simulink model "Controller"  (R2017b)
settings: Solver=VariableStepAuto  StartTime=0.0  StopTime=200  RelTol=1e-3
settings Model: Creator=Kris  LastModifiedBy=Kris

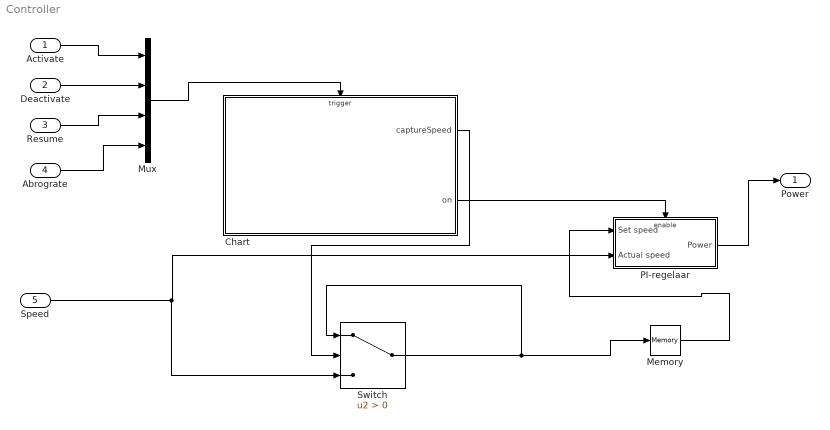
== system Controller ==
  Activate : Inport
  Deactivate : Inport  Port=2
  Resume : Inport  Port=3
  Abrograte : Inport  Port=4
  Speed : Inport  Port=5
  Chart : Stateflow chart  TreatAsAtomicUnit=on
  Memory : Memory
  Mux : Mux
  "PI-regelaar " : Subsystem
  Switch : Switch  Criteria=u2 > Threshold
  Power : Outport
  wires:
  Resume/1 -> Mux/3
  Speed/1 -> Switch/3, "PI-regelaar "/2(Actual speed)
  Chart/2(on) -> "PI-regelaar "/Enable
  Memory/1 -> "PI-regelaar "/1(Set speed)
  Mux/1 -> Chart/Trigger
  Deactivate/1 -> Mux/2
  Chart/1(captureSpeed) -> Switch/2
  "PI-regelaar "/1(Power) -> Power/1
  Abrograte/1 -> Mux/4
  Activate/1 -> Mux/1
  Switch/1 -> Memory/1, Switch/1

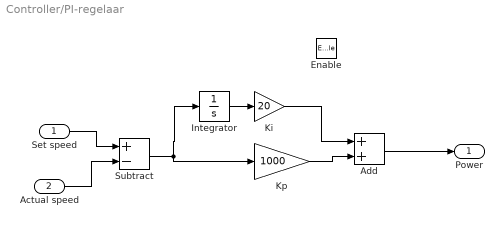
== system Controller/PI-regelaar  ==
  Set speed : Inport
  Actual speed : Inport  Port=2
  Enable : EnablePort
  Add : Sum
  Integrator : Integrator
  Ki : Gain  Gain=20
  Kp : Gain  Gain=1000
  Subtract : Sum  Inputs=+-
  Power : Outport
  wires:
  Kp/1 -> Add/2
  Ki/1 -> Add/1
  Actual speed/1 -> Subtract/2
  Subtract/1 -> Kp/1, Integrator/1
  Set speed/1 -> Subtract/1
  Add/1 -> Power/1
  Integrator/1 -> Ki/1

== stateflow chart Controller/Chart ==
  settings: executeAtInitialization=1
  state StateOff
    entry: on = 0;
    captureSpeed = 0;
  state StateOn
    entry: on = 1
    captureSpeed =1
  state stateSuspended
    entry: on = 0
    captureSpeed = 1;
  (default) -> StateOff
  StateOn -> StateOff [order 2] : deactivate
  stateSuspended -> StateOff [order 2] : deactivate
  StateOff -> StateOn : activate
  StateOn -> stateSuspended [order 1] : abrogate
  stateSuspended -> StateOn [order 1] : resume
  data: captureSpeed output; on output
  events: activate input RISING_EDGE_EVENT; deactivate input RISING_EDGE_EVENT; resume input RISING_EDGE_EVENT; abrogate input RISING_EDGE_EVENT
